simulink model "detect_fall_test"  (Simulink 8.4)
settings: Solver=ode45  StartTime=0.0  StopTime=10.0  RelTol=1e-3
libraries: simulink x8
settings Model: Creator=arnaud  LastModifiedBy=arnaud
settings DataIOCC: SaveFormat=StructureWithTime

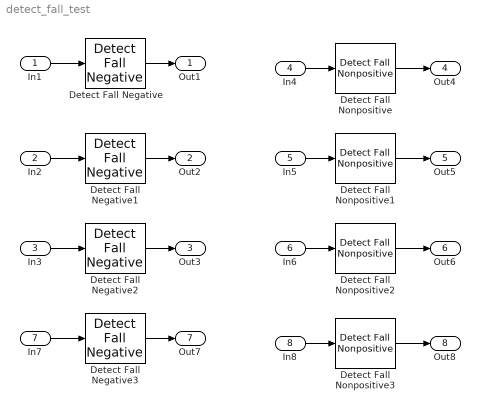
== system detect_fall_test ==
  In1 : Inport  PortDimensions=1
  In2 : Inport  Port=2  PortDimensions=5
  In3 : Inport  Port=3  OutDataTypeStr=int8  PortDimensions=[2 3]
  In4 : Inport  Port=4  PortDimensions=1
  In5 : Inport  Port=5  PortDimensions=5
  In6 : Inport  Port=6  OutDataTypeStr=int8  PortDimensions=[2 3]
  In7 : Inport  Port=7  OutDataTypeStr=boolean  PortDimensions=1
  In8 : Inport  Port=8  OutDataTypeStr=boolean  PortDimensions=1
  Detect Fall Negative{,1..3} (4 alike) : simulink/Logic and Bit Operations/Detect Fall Negative  vinit=0  InputProcessing=Inherited  OutDataTypeStr=boolean
  Detect Fall Nonpositive{,1..3} (4 alike) : simulink/Logic and Bit Operations/Detect Fall Nonpositive  vinit=0  InputProcessing=Inherited  OutDataTypeStr=boolean
  Out1 : Outport
  Out2 : Outport  Port=2
  Out3 : Outport  Port=3
  Out4 : Outport  Port=4
  Out5 : Outport  Port=5
  Out6 : Outport  Port=6
  Out7 : Outport  Port=7
  Out8 : Outport  Port=8
  wires:
  Detect Fall Negative/1 -> Out1/1
  In1/1 -> Detect Fall Negative/1
  Detect Fall Negative1/1 -> Out2/1
  In2/1 -> Detect Fall Negative1/1
  Detect Fall Negative2/1 -> Out3/1
  In3/1 -> Detect Fall Negative2/1
  In4/1 -> Detect Fall Nonpositive/1
  In5/1 -> Detect Fall Nonpositive1/1
  In6/1 -> Detect Fall Nonpositive2/1
  Detect Fall Nonpositive/1 -> Out4/1
  Detect Fall Nonpositive1/1 -> Out5/1
  Detect Fall Nonpositive2/1 -> Out6/1
  Detect Fall Negative3/1 -> Out7/1
  In7/1 -> Detect Fall Negative3/1
  In8/1 -> Detect Fall Nonpositive3/1
  Detect Fall Nonpositive3/1 -> Out8/1
